simulink model "MATLAB_TEST"  (R2019b)
settings: Solver=FixedStepDiscrete  StartTime=0  StopTime=50  FixedStep=0.0025  RelTol=1e-3
undefined symbols (not defined in the file): BCM_COM_PROC_P20, BCM_COM_PROC_P20_SFW_R2018b, BCM_COM_PROC_P2_5, BCM_COM_PROC_P2_5_SFW_R2018b, BCM_COM_PROC_P5, BCM_COM_PROC_P5_SFW_R2018b, BCMA_ACCU_PT_Conf_Flt, BCMA_ACCU_PT_Unconf_Flt, BCMA_Antiskid_Off_Sanction, BCMA_Avionics_Conf_Flt, BCMA_BCM_CCDL_Conf_Flt, BCMA_BCM_CCDL_Unconf_Flt, BCMA_BCM_DBCU_INHIBITION_Conf_Flt, BCMA_BCM_DBCU_INHIBITION_Unconf_Flt, BCMA_BCP_ALT_Disp_Sw_Conf_Flt, BCMA_BCP_ALT_Disp_Sw_Unconf_Flt, BCMA_BCP_ALT_SW_ON_CMD_Conf_Flt, BCMA_BCP_ALT_SW_ON_CMD_Unconf_Flt, BCMA_BCP_PARK_OFF_SW_CMD_Conf_Flt, BCMA_BCP_PARK_OFF_SW_CMD_Unconf_Flt, BCMA_CF_BSELV_JCL, BCMA_CF_BSELV_JOP, BCMA_CF_BSELV_OC, BCMA_CF_BSELV_SC, BCMA_CF_LH_SV_JCL, BCMA_CF_LH_SV_JOP, BCMA_CF_LH_SV_OC, BCMA_CF_LH_SV_SC, BCMA_CF_PARK_BRK, BCMA_CF_RESIDUAL_PRESS, BCMA_CF_RH_SV_JCL, BCMA_CF_RH_SV_JOP, BCMA_CF_RH_SV_OC, BCMA_CF_RH_SV_SC, BCMA_CF_SELV_JCL, BCMA_CF_SELV_JOP, BCMA_CF_SELV_OC, BCMA_CF_SELV_SC, BCMA_CF_SV_DRIFT, BCMA_DBCU_ALT_MODE_Conf_Flt, BCMA_DBCU_ALT_MODE_Unconf_Flt, BCMA_DBCU_BRK_ORDER_FAIL_Conf_Flt, BCMA_DBCU_BRK_ORDER_FAIL_Unconf_Flt, BCMA_DBCU_Conf_Flt, BCMA_DBCU_DISPATCH_SW_ON_Conf_Flt, BCMA_DBCU_DISPATCH_SW_ON_Unconf_Flt, BCMA_DBCU_FAILED_Conf_Flt, BCMA_DBCU_FAILED_Unconf_Flt, BCMA_DFCS1_Capsule_Validity, BCMA_DFCS1_Label202_Corrupted, BCMA_DFCS1_Label202_Not_Refreshed, BCMA_DFCS1_Label204_Corrupted, BCMA_DFCS1_Label204_Not_Refreshed, BCMA_DFCS1_Label205_Corrupted, BCMA_DFCS1_Label205_Not_Refreshed, BCMA_DFCS1_Label206_Corrupted, BCMA_DFCS1_Label206_Not_Refreshed, BCMA_DFCS1_Label207_Corrupted, BCMA_DFCS1_Label207_Not_Refreshed, BCMA_DFCS3_Capsule_Validity ... (+762)
libraries: simulink x73, lib_MBD_Control x5
(part 12 of 16)

== system MATLAB_TEST/AVIONICS/Brake_Control_Module_Side_A/BCSA Controller CP/BCM_COM_PROC_P2_5/BCM_COM_PROC_P2_5 ==
  V_BCM_COM_Tacho_Acq_W12 : Inport
  V_BCM_COM_Tacho_Unconf_Flt_W12 : Inport  Port=2
  V_BCM_COM_Tacho_Conf_Flt_W12 : Inport  Port=3
  V_BCM_COM_Tacho_Acq_W34 : Inport  Port=4
  V_BCM_COM_Tacho_Unconf_Flt_W34 : Inport  Port=5
  V_BCM_COM_Tacho_Conf_Flt_W34 : Inport  Port=6
  V_BCM_COM_Whl_LP_AS_Curr_Order_W12 : Inport  Port=7
  V_BCM_COM_Press_Cmd_Rate_Lim : Inport  Port=8
  V_BCM_COM_Whl_LP_AS_Curr_Order_W34 : Inport  Port=9
  V_BCM_COM_Global_Reference_Spd : Inport  Port=10
  V_BCM_COM_Wheels_Global_Spun_Up_Ste : Inport  Port=11
  BCM_Tuning : Inport  Port=12
  BCM_COM_PROC_P2_5 : S-Function  FunctionName=BCM_COM_PROC_P2_5_SFCT  SFunctionModules=|  SFunctionDeploymentMode=off  EnableBusSupport=off
      | BCM_COM_PROC_P2_5
      | BCM_COM_PROC_P2_5_SFCT
      | AC_Accel_Computation
      | FilteredWheelSpeed
      | ComputeAcqTachoWheelSpeed
      | ComputeTachometerError
      | ComputeFilteredWheelSpeed
      | ComputeRateLimitedWheelSpeed
      | ComputeWheelSpeedPreFiltering
      | F_ASLIB_10
      | F_Interpolate_ASLIB
      | DERIV_ASLIB
      | Filter_Wheel_Speeds_Noise
      | F_WHEELSPEED_FILTERING_BCS_SCM_IWS_C1
      | IND_FilteredWheelSpeed_SCM_IWS_C1
      | ComputeRateLimitedWheelSpeed_SCM_IWS_C1
      | ComputeTachometerError_SCM_IWS_C1
      | ComputeAsFilteredWheelSpeed_SCM_IWS_C1
      | PBS1_ASLIB
      | ComputeAntiskidFilterTimeConstant_SCM_IWS_C1
      | LIM_ASLIB
      | ComputeFilteredWheelSpeed_SCM_IWS_C1
      | FILT_ASLIB
      | ComputeWheelSpeedPreFiltering_SCM_IWS_C1
      | MIN_ASLIB_float32
      | MAX_ASLIB_float32
      | MINMAX4_ASLIB_float32
      | ComputeAcqTachoWheelSpeed_SCM_IWS_C1
      | MEM_ASLIB_float32
      | Consolidate_Wheel_Speeds
      | F_WHEEL_SPEED_CONSOLIDATION_BCS_SCM_WSC_C1
      | ComputeWheelSpeedConsoFunction_SCM_WSC_C1
      | ComputeWheelSpeedConso_SCM_WSC_C1
      | AIG4_ASLIB_float32
      | ComputeTachometerValidity_SCM_WSC_C1
      | BCM_COM_PROC_P2_5_KCG66_kcg_types
      | BCM_COM_PROC_P2_5_KCG66_kcg_consts
      | BCM_COM_PROC_P2_5_KCG66_kcg_consts
  DTC{1,4,7..10} (6 alike) : DataTypeConversion  OutDataTypeStr=single  SaturateOnIntegerOverflow=on  RndMeth=Zero
  DTC{2..3,5..6,11} (5 alike) : DataTypeConversion  OutDataTypeStr=boolean  SaturateOnIntegerOverflow=on  RndMeth=Zero
  Prb_AntiskidFilterTimeConstant : Terminator
  Prb_AntiskidFilterTimeConstant (1) : Terminator
  Prb_AntiskidFilterTimeConstant (2) : Terminator
  Prb_AntiskidFilterTimeConstant (3) : Terminator
  Prb_FilteredWheelSpeedAverage : Terminator
  Prb_FilteredWheelSpeedAverage (1) : Terminator
  Prb_FilteredWheelSpeedAverage (2) : Terminator
  Prb_FilteredWheelSpeedAverage (3) : Terminator
  Prb_RateLimitedWheelSpeed : Terminator
  Prb_RateLimitedWheelSpeed (1) : Terminator
  Prb_RateLimitedWheelSpeed (2) : Terminator
  Prb_RateLimitedWheelSpeed (3) : Terminator
  Prb_TachometerError : Terminator
  Prb_TachometerError (1) : Terminator
  Prb_TachometerError (2) : Terminator
  Prb_TachometerError (3) : Terminator
  Prb_WheelSpeed : Terminator
  Prb_WheelSpeed (1) : Terminator
  Prb_WheelSpeed (2) : Terminator
  Prb_WheelSpeed (3) : Terminator
  Prb_WheelSpeedAverage : Terminator
  Prb_WheelSpeedAverage (1) : Terminator
  Prb_WheelSpeedAverage (2) : Terminator
  Prb_WheelSpeedAverage (3) : Terminator
  Prb_WheelSpeedMax4 : Terminator
  Prb_WheelSpeedMax4 (1) : Terminator
  Prb_WheelSpeedMax4 (2) : Terminator
  Prb_WheelSpeedMax4 (3) : Terminator
  Prb_WheelSpeedMin4 : Terminator
  Prb_WheelSpeedMin4 (1) : Terminator
  Prb_WheelSpeedMin4 (2) : Terminator
  Prb_WheelSpeedMin4 (3) : Terminator
  Prb_WhlSpdIntermediate : Terminator
  Prb_WhlSpdIntermediate (1) : Terminator
  Prb_WhlSpdIntermediate (2) : Terminator
  Prb_WhlSpdIntermediate (3) : Terminator
  Subsystem : Subsystem
  v_BCM_COM_Press_Cmd_Rate_Lim_W12 : Terminator
  v_BCM_COM_Press_Cmd_Rate_Lim_W34 : Terminator
  V_BCM_COM_Wheel_Speed_Cons_W12 : Outport
  V_BCM_COM_Wheel_Speed_W12 : Outport  Port=2
  V_BCM_COM_Wheel_Speed_Val_W12 : Outport  Port=3
  V_BCM_COM_Wheel_Speed_Cons_W34 : Outport  Port=4
  V_BCM_COM_Wheel_Speed_W34 : Outport  Port=5
  V_BCM_COM_Wheel_Speed_Val_W34 : Outport  Port=6
  V_BCM_COM_Whl_Filt_Spd_For_AS_W12 : Outport  Port=7
  V_BCM_COM_Wheel_Filtered_Speed_W12 : Outport  Port=8
  V_BCM_COM_Min_Last_8_Whl_Spd_W12 : Outport  Port=9
  V_BCM_COM_Max_Last_8_Whl_Spd_W12 : Outport  Port=10
  V_BCM_COM_Whl_Filt_Spd_For_AS_W34 : Outport  Port=11
  V_BCM_COM_Wheel_Filtered_Speed_W34 : Outport  Port=12
  V_BCM_COM_Min_Last_8_Whl_Spd_W34 : Outport  Port=13
  V_BCM_COM_Max_Last_8_Whl_Spd_W34 : Outport  Port=14
  V_BCM_COM_DCL_Acc : Outport  Port=15
  V_BCM_COM_CT_BCS_WS_First_Filter : Outport  Port=16
  wires:
  V_BCM_COM_Tacho_Acq_W12/1 -> DTC1/1
  DTC1/1 -> BCM_COM_PROC_P2_5/1
  V_BCM_COM_Tacho_Unconf_Flt_W12/1 -> DTC2/1
  DTC2/1 -> BCM_COM_PROC_P2_5/2
  V_BCM_COM_Tacho_Conf_Flt_W12/1 -> DTC3/1
  DTC3/1 -> BCM_COM_PROC_P2_5/3
  V_BCM_COM_Tacho_Acq_W34/1 -> DTC4/1
  DTC4/1 -> BCM_COM_PROC_P2_5/4
  V_BCM_COM_Tacho_Unconf_Flt_W34/1 -> DTC5/1
  DTC5/1 -> BCM_COM_PROC_P2_5/5
  V_BCM_COM_Tacho_Conf_Flt_W34/1 -> DTC6/1
  DTC6/1 -> BCM_COM_PROC_P2_5/6
  V_BCM_COM_Whl_LP_AS_Curr_Order_W12/1 -> DTC7/1
  DTC7/1 -> BCM_COM_PROC_P2_5/7
  V_BCM_COM_Press_Cmd_Rate_Lim/1 -> DTC8/1
  DTC8/1 -> BCM_COM_PROC_P2_5/8
  V_BCM_COM_Whl_LP_AS_Curr_Order_W34/1 -> DTC9/1
  DTC9/1 -> BCM_COM_PROC_P2_5/9
  V_BCM_COM_Global_Reference_Spd/1 -> DTC10/1
  DTC10/1 -> BCM_COM_PROC_P2_5/10
  V_BCM_COM_Wheels_Global_Spun_Up_Ste/1 -> DTC11/1
  DTC11/1 -> BCM_COM_PROC_P2_5/11
  BCM_COM_PROC_P2_5/1 -> V_BCM_COM_Wheel_Speed_Cons_W12/1
  BCM_COM_PROC_P2_5/2 -> V_BCM_COM_Wheel_Speed_W12/1
  BCM_COM_PROC_P2_5/3 -> V_BCM_COM_Wheel_Speed_Val_W12/1
  BCM_COM_PROC_P2_5/4 -> V_BCM_COM_Wheel_Speed_Cons_W34/1
  BCM_COM_PROC_P2_5/5 -> V_BCM_COM_Wheel_Speed_W34/1
  BCM_COM_PROC_P2_5/6 -> V_BCM_COM_Wheel_Speed_Val_W34/1
  BCM_COM_PROC_P2_5/7 -> V_BCM_COM_Whl_Filt_Spd_For_AS_W12/1
  BCM_COM_PROC_P2_5/8 -> V_BCM_COM_Wheel_Filtered_Speed_W12/1
  BCM_COM_PROC_P2_5/9 -> V_BCM_COM_Min_Last_8_Whl_Spd_W12/1
  BCM_COM_PROC_P2_5/10 -> V_BCM_COM_Max_Last_8_Whl_Spd_W12/1
  BCM_COM_PROC_P2_5/11 -> V_BCM_COM_Whl_Filt_Spd_For_AS_W34/1
  BCM_COM_PROC_P2_5/12 -> V_BCM_COM_Wheel_Filtered_Speed_W34/1
  BCM_COM_PROC_P2_5/13 -> V_BCM_COM_Min_Last_8_Whl_Spd_W34/1
  BCM_COM_PROC_P2_5/14 -> V_BCM_COM_Max_Last_8_Whl_Spd_W34/1
  BCM_COM_PROC_P2_5/15 -> V_BCM_COM_DCL_Acc/1
  BCM_COM_PROC_P2_5/16 -> V_BCM_COM_CT_BCS_WS_First_Filter/1
  BCM_COM_PROC_P2_5/17 -> Prb_WheelSpeed/1  "Prb_WheelSpeed_1_BCMA"
  BCM_COM_PROC_P2_5/18 -> Prb_WhlSpdIntermediate/1  "Prb_WhlSpdIntermediate_1_BCMA"
  BCM_COM_PROC_P2_5/19 -> Prb_WheelSpeedMin4/1  "Prb_WheelSpeedMin4_1_BCMA"
  BCM_COM_PROC_P2_5/20 -> Prb_WheelSpeedMax4/1  "Prb_WheelSpeedMax4_1_BCMA"
  BCM_COM_PROC_P2_5/21 -> Prb_WheelSpeedAverage/1  "Prb_WheelSpeedAverage_1_BCMA"
  BCM_COM_PROC_P2_5/22 -> Prb_FilteredWheelSpeedAverage/1  "Prb_FilteredWheelSpeedAverage_1_BCMA"
  BCM_COM_PROC_P2_5/23 -> Prb_TachometerError/1  "Prb_TachometerError_1_BCMA"
  BCM_COM_PROC_P2_5/24 -> Prb_RateLimitedWheelSpeed/1  "Prb_RateLimitedWheelSpeed_1_BCMA"
  BCM_COM_PROC_P2_5/25 -> Prb_AntiskidFilterTimeConstant/1  "Prb_AntiskidFilterTimeConstant_1_BCMA"
  BCM_COM_PROC_P2_5/26 -> Prb_WheelSpeed (1)/1  "Prb_WheelSpeed_2_BCMA"
  BCM_COM_PROC_P2_5/27 -> Prb_WhlSpdIntermediate (1)/1  "Prb_WhlSpdIntermediate_2_BCMA"
  BCM_COM_PROC_P2_5/28 -> Prb_WheelSpeedMin4 (1)/1  "Prb_WheelSpeedMin4_2_BCMA"
  BCM_COM_PROC_P2_5/29 -> Prb_WheelSpeedMax4 (1)/1  "Prb_WheelSpeedMax4_2_BCMA"
  BCM_COM_PROC_P2_5/30 -> Prb_WheelSpeedAverage (1)/1  "Prb_WheelSpeedAverage_2_BCMA"
  BCM_COM_PROC_P2_5/31 -> Prb_FilteredWheelSpeedAverage (1)/1  "Prb_FilteredWheelSpeedAverage_2_BCMA"
  BCM_COM_PROC_P2_5/32 -> Prb_TachometerError (1)/1  "Prb_TachometerError_2_BCMA"
  BCM_COM_PROC_P2_5/33 -> Prb_RateLimitedWheelSpeed (1)/1  "Prb_RateLimitedWheelSpeed_2_BCMA"
  BCM_COM_PROC_P2_5/34 -> Prb_AntiskidFilterTimeConstant (1)/1  "Prb_AntiskidFilterTimeConstant_2_BCMA"
  BCM_COM_PROC_P2_5/35 -> Prb_WheelSpeed (2)/1  "Prb_WheelSpeed_3_BCMA"
  BCM_COM_PROC_P2_5/36 -> Prb_WhlSpdIntermediate (2)/1  "Prb_WhlSpdIntermediate_3_BCMA"
  BCM_COM_PROC_P2_5/37 -> Prb_WheelSpeedMin4 (2)/1  "Prb_WheelSpeedMin4_3_BCMA"
  BCM_COM_PROC_P2_5/38 -> Prb_WheelSpeedMax4 (2)/1  "Prb_WheelSpeedMax4_3_BCMA"
  BCM_COM_PROC_P2_5/39 -> Prb_WheelSpeedAverage (2)/1  "Prb_WheelSpeedAverage_3_BCMA"
  BCM_COM_PROC_P2_5/40 -> Prb_FilteredWheelSpeedAverage (2)/1  "Prb_FilteredWheelSpeedAverage_3_BCMA"
  BCM_COM_PROC_P2_5/41 -> Prb_TachometerError (2)/1  "Prb_TachometerError_3_BCMA"
  BCM_COM_PROC_P2_5/42 -> Prb_RateLimitedWheelSpeed (2)/1  "Prb_RateLimitedWheelSpeed_3_BCMA"
  BCM_COM_PROC_P2_5/43 -> Prb_AntiskidFilterTimeConstant (2)/1  "Prb_AntiskidFilterTimeConstant_3_BCMA"
  BCM_COM_PROC_P2_5/44 -> Prb_WheelSpeed (3)/1  "Prb_WheelSpeed_4_BCMA"
  BCM_COM_PROC_P2_5/45 -> Prb_WhlSpdIntermediate (3)/1  "Prb_WhlSpdIntermediate_4_BCMA"
  BCM_COM_PROC_P2_5/46 -> Prb_WheelSpeedMin4 (3)/1  "Prb_WheelSpeedMin4_4_BCMA"
  BCM_COM_PROC_P2_5/47 -> Prb_WheelSpeedMax4 (3)/1  "Prb_WheelSpeedMax4_4_BCMA"
  BCM_COM_PROC_P2_5/48 -> Prb_WheelSpeedAverage (3)/1  "Prb_WheelSpeedAverage_4_BCMA"
  BCM_COM_PROC_P2_5/49 -> Prb_FilteredWheelSpeedAverage (3)/1  "Prb_FilteredWheelSpeedAverage_4_BCMA"
  BCM_COM_PROC_P2_5/50 -> Prb_TachometerError (3)/1  "Prb_TachometerError_4_BCMA"
  BCM_COM_PROC_P2_5/51 -> Prb_RateLimitedWheelSpeed (3)/1  "Prb_RateLimitedWheelSpeed_4_BCMA"
  BCM_COM_PROC_P2_5/52 -> Prb_AntiskidFilterTimeConstant (3)/1  "Prb_AntiskidFilterTimeConstant_4_BCMA"
  BCM_COM_PROC_P2_5/53 -> v_BCM_COM_Press_Cmd_Rate_Lim_W12/1  "v_BCM_COM_Press_Cmd_Rate_Lim_W12_1_BCMA"
  BCM_COM_PROC_P2_5/54 -> v_BCM_COM_Press_Cmd_Rate_Lim_W34/1  "v_BCM_COM_Press_Cmd_Rate_Lim_W34_1_BCMA"
  BCM_Tuning/1 -> Subsystem/1(In1)
  Subsystem/1(Out1) -> BCM_COM_PROC_P2_5/12
  Subsystem/2(Out2) -> BCM_COM_PROC_P2_5/13
  Subsystem/3(Out3) -> BCM_COM_PROC_P2_5/14
  Subsystem/4(Out4) -> BCM_COM_PROC_P2_5/15
  Subsystem/5(Out5) -> BCM_COM_PROC_P2_5/16
  Subsystem/6(Out6) -> BCM_COM_PROC_P2_5/17
  Subsystem/7(Out7) -> BCM_COM_PROC_P2_5/18
  Subsystem/8(Out8) -> BCM_COM_PROC_P2_5/19
  Subsystem/9(Out9) -> BCM_COM_PROC_P2_5/20
  Subsystem/10(Out10) -> BCM_COM_PROC_P2_5/21
  Subsystem/11(Out11) -> BCM_COM_PROC_P2_5/22
  Subsystem/12(Out12) -> BCM_COM_PROC_P2_5/23
  Subsystem/13(Out13) -> BCM_COM_PROC_P2_5/24
  Subsystem/14(Out14) -> BCM_COM_PROC_P2_5/25
  Subsystem/15(Out15) -> BCM_COM_PROC_P2_5/26
  Subsystem/16(Out16) -> BCM_COM_PROC_P2_5/27
  Subsystem/17(Out17) -> BCM_COM_PROC_P2_5/28
  Subsystem/18(Out18) -> BCM_COM_PROC_P2_5/29
  Subsystem/19(Out19) -> BCM_COM_PROC_P2_5/30
  Subsystem/20(Out20) -> BCM_COM_PROC_P2_5/31
  Subsystem/21(Out21) -> BCM_COM_PROC_P2_5/32
  Subsystem/22(Out22) -> BCM_COM_PROC_P2_5/33
  Subsystem/23(Out23) -> BCM_COM_PROC_P2_5/34
  Subsystem/24(Out24) -> BCM_COM_PROC_P2_5/35
  Subsystem/25(Out25) -> BCM_COM_PROC_P2_5/36

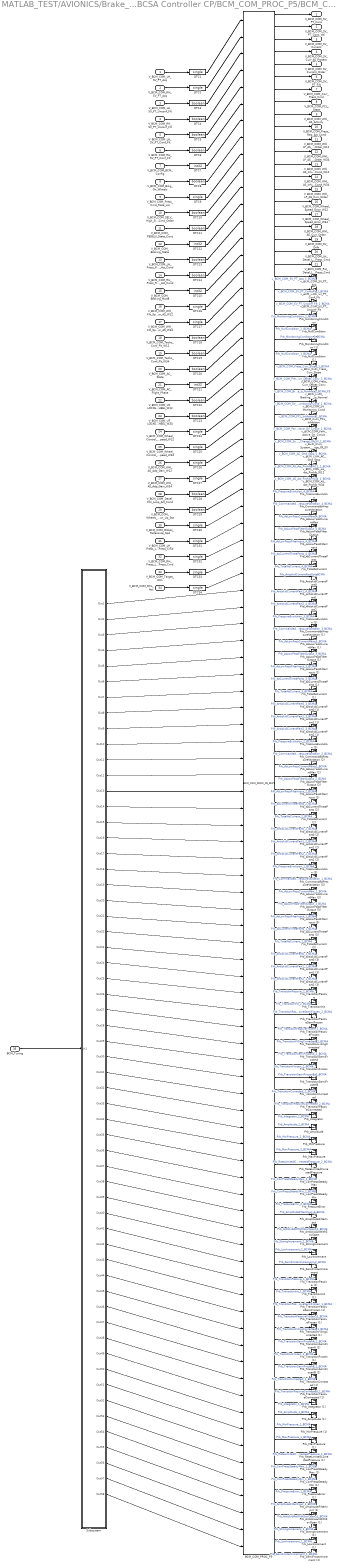
== system MATLAB_TEST/AVIONICS/Brake_Control_Module_Side_A/BCSA Controller CP/BCM_COM_PROC_P5/BCM_COM_PROC_P5 ==
  V_BCM_COM_LH_SV_PT_Acq : Inport
  V_BCM_COM_RH_SV_PT_Acq : Inport  Port=2
  V_BCM_COM_LH_SV_PT_Unconf_Flt : Inport  Port=3
  V_BCM_COM_RH_SV_PT_Unconf_Flt : Inport  Port=4
  V_BCM_COM_LH_SV_PT_Conf_Flt : Inport  Port=5
  V_BCM_COM_RH_SV_PT_Conf_Flt : Inport  Port=6
  V_BCM_COM_BCM_Config : Inport  Port=7
  V_BCM_COM_Brkg_On_Wheels : Inport  Port=8
  V_BCM_COM_Press_Cmd_Rate_Lim : Inport  Port=9
  V_BCM_COM_SELV_High_Side_Cmd_Order : Inport  Port=10
  V_BCM_COM_PBSELV_State_Cons : Inport  Port=11
  V_BCM_COM_Braking_State : Inport  Port=12
  V_BCM_COM_LH_Press_Reg_FT_Act_Cond : Inport  Port=13
  V_BCM_COM_RH_Press_Reg_FT_Act_Cond : Inport  Port=14
  V_BCM_COM_Braking_Mode : Inport  Port=15
  V_BCM_COM_Whl_Filt_Spd_For_AS_W12 : Inport  Port=16
  V_BCM_COM_Whl_Filt_Spd_For_AS_W34 : Inport  Port=17
  V_BCM_COM_Tacho_Conf_Flt_W12 : Inport  Port=18
  V_BCM_COM_Tacho_Conf_Flt_W34 : Inport  Port=19
  V_BCM_COM_AC_State : Inport  Port=20
  V_BCM_COM_AC_Flight_Phase : Inport  Port=21
  V_BCM_COM_UF_LOCKED_WHEEL_W12 : Inport  Port=22
  V_BCM_COM_UF_LOCKED_WHEEL_W34 : Inport  Port=23
  V_BCM_COM_Wheel_Control_Speed_W12 : Inport  Port=24
  V_BCM_COM_Wheel_Control_Speed_W34 : Inport  Port=25
  V_BCM_COM_Whl_AS_Adp_Gain_W12 : Inport  Port=26
  V_BCM_COM_Whl_AS_Adp_Gain_W34 : Inport  Port=27
  V_BCM_COM_Decel_Ctrl_Loop_Act_Cond : Inport  Port=28
  V_BCM_COM_Wheels_Global_Spun_Up_Ste : Inport  Port=29
  V_BCM_COM_Global_Reference_Spd : Inport  Port=30
  V_BCM_COM_LH_Press_Law_Brkg_Press_Cmd : Inport  Port=31
  V_BCM_COM_RH_Press_Law_Brkg_Press_Cmd : Inport  Port=32
  V_BCM_COM_Target_DCL : Inport  Port=33
  V_BCM_COM_DCL_Acc : Inport  Port=34
  BCM_Tuning : Inport  Port=35
  BCM_COM_PROC_P5 : S-Function  FunctionName=BCM_COM_PROC_P5_SFCT  SFunctionModules=<binary blob, 3799 chars, not shown>  SFunctionDeploymentMode=off  EnableBusSupport=off
  DTC{1..2,9,16..17,24..27,30..34} (14 alike) : DataTypeConversion  OutDataTypeStr=single  SaturateOnIntegerOverflow=on  RndMeth=Zero
  DTC{3..6,8,10..11,13..14,18..20,22..23,28..29} (16 alike) : DataTypeConversion  OutDataTypeStr=boolean  SaturateOnIntegerOverflow=on  RndMeth=Zero
  DTC{7,12,15,21} (4 alike) : DataTypeConversion  OutDataTypeStr=int32  SaturateOnIntegerOverflow=on  RndMeth=Zero
  Prb_Amplitude : Terminator
  Prb_Amplitude (1) : Terminator
  Prb_AmplitudeFilterInput : Terminator
  Prb_AmplitudeFilterInput (1) : Terminator
  Prb_AntiskidActWithSovOpen : Terminator
  Prb_AntiskidActWithSovOpen (1) : Terminator
  Prb_AntiskidCurrentPart0 : Terminator
  Prb_AntiskidCurrentPart0 (1) : Terminator
  Prb_AntiskidCurrentPart0 (2) : Terminator
  Prb_AntiskidCurrentPart0 (3) : Terminator
  Prb_AntiskidCurrentPart1 : Terminator
  Prb_AntiskidCurrentPart1 (1) : Terminator
  Prb_AntiskidCurrentPart1 (2) : Terminator
  Prb_AntiskidCurrentPart1 (3) : Terminator
  Prb_AntiskidCurrentPart2 : Terminator
  Prb_AntiskidCurrentPart2 (1) : Terminator
  Prb_AntiskidCurrentPart2 (2) : Terminator
  Prb_AntiskidCurrentPart2 (3) : Terminator
  Prb_AsCurrentThreeParts : Terminator
  Prb_AsCurrentThreeParts (1) : Terminator
  Prb_AsCurrentThreeParts (2) : Terminator
  Prb_AsCurrentThreeParts (3) : Terminator
  Prb_AsLowPassCurrentMax : Terminator
  Prb_AsLowPassCurrentMax (1) : Terminator
  Prb_AsLowPassCurrentMax (2) : Terminator
  Prb_AsLowPassCurrentMax (3) : Terminator
  Prb_AsLowPassFilterInput : Terminator
  Prb_AsLowPassFilterInput (1) : Terminator
  Prb_AsLowPassFilterInput (2) : Terminator
  Prb_AsLowPassFilterInput (3) : Terminator
  Prb_AsLowPassFilterOutput : Terminator
  Prb_AsLowPassFilterOutput (1) : Terminator
  Prb_AsLowPassFilterOutput (2) : Terminator
  Prb_AsLowPassFilterOutput (3) : Terminator
  Prb_CommandedPressureVariation : Terminator
  Prb_CommandedPressureVariation (1) : Terminator
  Prb_CommandedPressureVariation (2) : Terminator
  Prb_CommandedPressureVariation (3) : Terminator
  Prb_CorrPressSteadyMax : Terminator
  Prb_CorrPressSteadyMax (1) : Terminator
  Prb_CorrPressSteadyMin : Terminator
  Prb_CorrPressSteadyMin (1) : Terminator
  Prb_Integrator : Terminator
  Prb_Integrator (1) : Terminator
  Prb_LowIncrement : Terminator
  Prb_LowIncrement (1) : Terminator
  Prb_MaxPressure : Terminator
  Prb_MaxPressure (1) : Terminator
  Prb_MinPressure : Terminator
  Prb_MinPressure (1) : Terminator
  Prb_MonitoringCondition : Terminator
  Prb_MonitoringCondition (1) : Terminator
  Prb_NullCondition : Terminator
  Prb_NullCondition (1) : Terminator
  Prb_PressureError : Terminator
  Prb_PressureError (1) : Terminator
  Prb_PressureEvolution : Terminator
  Prb_PressureEvolution (1) : Terminator
  Prb_PressureEvolution (2) : Terminator
  Prb_PressureEvolution (3) : Terminator
  Prb_RateLimitedCorrectedPressure : Terminator
  Prb_RateLimitedCorrectedPressure (1) : Terminator
  Prb_SemiFrozenIncrement : Terminator
  Prb_SemiFrozenIncrement (1) : Terminator
  Prb_StrongIncrement : Terminator
  Prb_StrongIncrement (1) : Terminator
  Prb_TotalAsCurrent : Terminator
  Prb_TotalAsCurrent (1) : Terminator
  Prb_TotalAsCurrent (2) : Terminator
  Prb_TotalAsCurrent (3) : Terminator
  Prb_TransitionCorrected : Terminator
  Prb_TransitionCorrected (1) : Terminator
  Prb_TransitionFillingCorrected : Terminator
  Prb_TransitionFillingCorrected (1) : Terminator
  Prb_TransitionFrozen : Terminator
  Prb_TransitionFrozen (1) : Terminator
  Prb_TransitionInit : Terminator
  Prb_TransitionInit (1) : Terminator
  Prb_TransitionPassive : Terminator
  Prb_TransitionPassive (1) : Terminator
  Prb_TransitionPassiveCorrrected : Terminator
  Prb_TransitionPassiveCorrrected (1) : Terminator
  Prb_TransitionPassiveFrozen : Terminator
  Prb_TransitionPassiveFrozen (1) : Terminator
  Prb_TransitionPassiveSemiFrozen : Terminator
  Prb_TransitionPassiveSemiFrozen (1) : Terminator
  Prb_TransitionSemiFrozenA : Terminator
  Prb_TransitionSemiFrozenA (1) : Terminator
  Prb_TransitionSemiFrozenB : Terminator
  Prb_TransitionSemiFrozenB (1) : Terminator
  Subsystem : Subsystem
  v_BCM_COM_AC_Gnd_Stop : Terminator
  v_BCM_COM_AS_Act_Prohib_W12 : Terminator
  v_BCM_COM_AS_Act_Prohib_W34 : Terminator
  v_BCM_COM_Braking_Ste_Is_Normal : Terminator
  v_BCM_COM_PCL_Inhibition : Terminator
  v_BCM_COM_Park_Active_On_Circuit : Terminator
  v_BCM_COM_Press_Curr_Offset_Conv : Terminator
  v_BCM_COM_Press_Curr_Slope : Terminator
  v_BCM_COM_SV_Monitoring_Cond : Terminator
  v_BCM_COM_SV_PT_Acq : Terminator
  v_BCM_COM_SV_PT_Conf_Flt : Terminator
  v_BCM_COM_SV_PT_Unconf_Flt : Terminator
  v_BCM_COM_System_In_Charge_Of_SV : Terminator
  V_BCM_COM_SV_PT_Cons : Outport
  V_BCM_COM_SV_PT_Cons_Val : Outport  Port=2
  V_BCM_COM_SV_Current : Outport  Port=3
  V_BCM_COM_SV_Curr_AS_Protect : Outport  Port=4
  V_BCM_COM_SV_Current_Order : Outport  Port=5
  V_BCM_COM_SV_PT_Filt : Outport  Port=6
  V_BCM_COM_Corr_Press_Cmd : Outport  Port=7
  V_BCM_COM_PCL_State : Outport  Port=8
  V_BCM_COM_Whl_AS_Activity : Outport  Port=9
  V_BCM_COM_Press_Reg_Act_Cond : Outport  Port=10
  V_BCM_COM_Whl_LP_AS_Curr_Order_W12 : Outport  Port=11
  V_BCM_COM_Whl_LP_AS_Curr_Order_W34 : Outport  Port=12
  V_BCM_COM_Whl_AS_Inhib_Cond_W12 : Outport  Port=13
  V_BCM_COM_Whl_AS_Inhib_Cond_W34 : Outport  Port=14
  V_BCM_COM_Whl_LP_AS_Curr_Order : Outport  Port=15
  V_BCM_COM_Wheel_Speed_Error_W12 : Outport  Port=16
  V_BCM_COM_Wheel_Speed_Error_W34 : Outport  Port=17
  V_BCM_COM_Whl_AS_Curr_Order : Outport  Port=18
  V_BCM_COM_SV_Drift : Outport  Port=19
  V_BCM_COM_LH_Decel_Law_Brkg_Press_Cmd : Outport  Port=20
  V_BCM_COM_RH_Decel_Law_Brkg_Press_Cmd : Outport  Port=21
  wires:
  BCM_COM_PROC_P5/124 -> Prb_SemiFrozenIncrement (1)/1  "Prb_SemiFrozenIncrement_1_BCMA"
  BCM_COM_PROC_P5/123 -> Prb_LowIncrement (1)/1  "Prb_LowIncrement_1_BCMA"
  BCM_COM_PROC_P5/122 -> Prb_StrongIncrement (1)/1  "Prb_StrongIncrement_1_BCMA"
  BCM_COM_PROC_P5/121 -> Prb_AntiskidActWithSovOpen (1)/1  "Prb_AntiskidActWithSovOpen_1_BCMA"
  BCM_COM_PROC_P5/120 -> Prb_AmplitudeFilterInput (1)/1  "Prb_AmplitudeFilterInput_1_BCMA"
  BCM_COM_PROC_P5/119 -> Prb_PressureError (1)/1  "Prb_PressureError_1_BCMA"
  BCM_COM_PROC_P5/118 -> Prb_CorrPressSteadyMin (1)/1  "Prb_CorrPressSteadyMin_1_BCMA"
  BCM_COM_PROC_P5/117 -> Prb_CorrPressSteadyMax (1)/1  "Prb_CorrPressSteadyMax_1_BCMA"
  BCM_COM_PROC_P5/116 -> Prb_RateLimitedCorrectedPressure (1)/1  "Prb_RateLimitedCorrectedPressure_1_BCMA"
  BCM_COM_PROC_P5/115 -> Prb_MaxPressure (1)/1  "Prb_MaxPressure_1_BCMA"
  BCM_COM_PROC_P5/114 -> Prb_MinPressure (1)/1  "Prb_MinPressure_1_BCMA"
  BCM_COM_PROC_P5/113 -> Prb_Amplitude (1)/1  "Prb_Amplitude_1_BCMA"
  BCM_COM_PROC_P5/112 -> Prb_Integrator (1)/1  "Prb_Integrator_1_BCMA"
  BCM_COM_PROC_P5/111 -> Prb_TransitionPassiveCorrrected (1)/1  "Prb_TransitionPassiveCorrrected_1_BCMA"
  BCM_COM_PROC_P5/110 -> Prb_TransitionCorrected (1)/1  "Prb_TransitionCorrected_1_BCMA"
  BCM_COM_PROC_P5/109 -> Prb_TransitionSemiFrozenB (1)/1  "Prb_TransitionSemiFrozenB_1_BCMA"
  BCM_COM_PROC_P5/108 -> Prb_TransitionFrozen (1)/1  "Prb_TransitionFrozen_1_BCMA"
  BCM_COM_PROC_P5/107 -> Prb_TransitionSemiFrozenA (1)/1  "Prb_TransitionSemiFrozenA_1_BCMA"
  BCM_COM_PROC_P5/106 -> Prb_TransitionFillingCorrected (1)/1  "Prb_TransitionFillingCorrected_1_BCMA"
  BCM_COM_PROC_P5/105 -> Prb_TransitionPassiveFrozen (1)/1  "Prb_TransitionPassiveFrozen_1_BCMA"
  BCM_COM_PROC_P5/104 -> Prb_TransitionPassiveSemiFrozen (1)/1  "Prb_TransitionPassiveSemiFrozen_1_BCMA"
  BCM_COM_PROC_P5/103 -> Prb_TransitionInit (1)/1  "Prb_TransitionInit_1_BCMA"
  BCM_COM_PROC_P5/102 -> Prb_TransitionPassive (1)/1  "Prb_TransitionPassive_1_BCMA"
  BCM_COM_PROC_P5/101 -> Prb_SemiFrozenIncrement/1  "Prb_SemiFrozenIncrement_2_BCMA"
  BCM_COM_PROC_P5/100 -> Prb_LowIncrement/1  "Prb_LowIncrement_2_BCMA"
  BCM_COM_PROC_P5/99 -> Prb_StrongIncrement/1  "Prb_StrongIncrement_2_BCMA"
  BCM_COM_PROC_P5/98 -> Prb_AntiskidActWithSovOpen/1  "Prb_AntiskidActWithSovOpen_2_BCMA"
  BCM_COM_PROC_P5/97 -> Prb_AmplitudeFilterInput/1  "Prb_AmplitudeFilterInput_2_BCMA"
  BCM_COM_PROC_P5/96 -> Prb_PressureError/1  "Prb_PressureError_2_BCMA"
  BCM_COM_PROC_P5/95 -> Prb_CorrPressSteadyMin/1  "Prb_CorrPressSteadyMin_2_BCMA"
  BCM_COM_PROC_P5/94 -> Prb_CorrPressSteadyMax/1  "Prb_CorrPressSteadyMax_2_BCMA"
  BCM_COM_PROC_P5/93 -> Prb_RateLimitedCorrectedPressure/1  "Prb_RateLimitedCorrectedPressure_2_BCMA"
  BCM_COM_PROC_P5/92 -> Prb_MaxPressure/1  "Prb_MaxPressure_2_BCMA"
  BCM_COM_PROC_P5/91 -> Prb_MinPressure/1  "Prb_MinPressure_2_BCMA"
  BCM_COM_PROC_P5/90 -> Prb_Amplitude/1  "Prb_Amplitude_2_BCMA"
  BCM_COM_PROC_P5/89 -> Prb_Integrator/1  "Prb_Integrator_2_BCMA"
  BCM_COM_PROC_P5/88 -> Prb_TransitionPassiveCorrrected/1  "Prb_TransitionPassiveCorrrected_2_BCMA"
  BCM_COM_PROC_P5/87 -> Prb_TransitionCorrected/1  "Prb_TransitionCorrected_2_BCMA"
  BCM_COM_PROC_P5/86 -> Prb_TransitionSemiFrozenB/1  "Prb_TransitionSemiFrozenB_2_BCMA"
  BCM_COM_PROC_P5/85 -> Prb_TransitionFrozen/1  "Prb_TransitionFrozen_2_BCMA"
  BCM_COM_PROC_P5/84 -> Prb_TransitionSemiFrozenA/1  "Prb_TransitionSemiFrozenA_2_BCMA"
  BCM_COM_PROC_P5/83 -> Prb_TransitionFillingCorrected/1  "Prb_TransitionFillingCorrected_2_BCMA"
  BCM_COM_PROC_P5/82 -> Prb_TransitionPassiveFrozen/1  "Prb_TransitionPassiveFrozen_2_BCMA"
  BCM_COM_PROC_P5/81 -> Prb_TransitionPassiveSemiFrozen/1  "Prb_TransitionPassiveSemiFrozen_2_BCMA"
  BCM_COM_PROC_P5/80 -> Prb_TransitionInit/1  "Prb_TransitionInit_2_BCMA"
  BCM_COM_PROC_P5/79 -> Prb_TransitionPassive/1  "Prb_TransitionPassive_2_BCMA"
  BCM_COM_PROC_P5/78 -> Prb_AntiskidCurrentPart2 (3)/1  "Prb_AntiskidCurrentPart2_1_BCMA"
  BCM_COM_PROC_P5/77 -> Prb_AntiskidCurrentPart1 (3)/1  "Prb_AntiskidCurrentPart1_1_BCMA"
  BCM_COM_PROC_P5/76 -> Prb_AntiskidCurrentPart0 (3)/1  "Prb_AntiskidCurrentPart0_1_BCMA"
  BCM_COM_PROC_P5/75 -> Prb_TotalAsCurrent (3)/1  "Prb_TotalAsCurrent_1_BCMA"
  BCM_COM_PROC_P5/74 -> Prb_AsCurrentThreeParts (3)/1  "Prb_AsCurrentThreeParts_1_BCMA"
  BCM_COM_PROC_P5/73 -> Prb_AsLowPassFilterInput (3)/1  "Prb_AsLowPassFilterInput_1_BCMA"
  BCM_COM_PROC_P5/72 -> Prb_AsLowPassFilterOutput (3)/1  "Prb_AsLowPassFilterOutput_1_BCMA"
  BCM_COM_PROC_P5/71 -> Prb_AsLowPassCurrentMax (3)/1  "Prb_AsLowPassCurrentMax_1_BCMA"
  BCM_COM_PROC_P5/70 -> Prb_CommandedPressureVariation (3)/1  "Prb_CommandedPressureVariation_1_BCMA"
  BCM_COM_PROC_P5/69 -> Prb_PressureEvolution (3)/1  "Prb_PressureEvolution_1_BCMA"
  BCM_COM_PROC_P5/68 -> Prb_AntiskidCurrentPart2 (2)/1  "Prb_AntiskidCurrentPart2_2_BCMA"
  BCM_COM_PROC_P5/67 -> Prb_AntiskidCurrentPart1 (2)/1  "Prb_AntiskidCurrentPart1_2_BCMA"
  BCM_COM_PROC_P5/66 -> Prb_AntiskidCurrentPart0 (2)/1  "Prb_AntiskidCurrentPart0_2_BCMA"
  BCM_COM_PROC_P5/65 -> Prb_TotalAsCurrent (2)/1  "Prb_TotalAsCurrent_2_BCMA"
  BCM_COM_PROC_P5/64 -> Prb_AsCurrentThreeParts (2)/1  "Prb_AsCurrentThreeParts_2_BCMA"
  BCM_COM_PROC_P5/63 -> Prb_AsLowPassFilterInput (2)/1  "Prb_AsLowPassFilterInput_2_BCMA"
  BCM_COM_PROC_P5/62 -> Prb_AsLowPassFilterOutput (2)/1  "Prb_AsLowPassFilterOutput_2_BCMA"
  BCM_COM_PROC_P5/61 -> Prb_AsLowPassCurrentMax (2)/1  "Prb_AsLowPassCurrentMax_2_BCMA"
  BCM_COM_PROC_P5/60 -> Prb_CommandedPressureVariation (2)/1  "Prb_CommandedPressureVariation_2_BCMA"
  BCM_COM_PROC_P5/59 -> Prb_PressureEvolution (2)/1  "Prb_PressureEvolution_2_BCMA"
  BCM_COM_PROC_P5/58 -> Prb_AntiskidCurrentPart2 (1)/1  "Prb_AntiskidCurrentPart2_3_BCMA"
  BCM_COM_PROC_P5/57 -> Prb_AntiskidCurrentPart1 (1)/1  "Prb_AntiskidCurrentPart1_3_BCMA"
  BCM_COM_PROC_P5/56 -> Prb_AntiskidCurrentPart0 (1)/1  "Prb_AntiskidCurrentPart0_3_BCMA"
  BCM_COM_PROC_P5/55 -> Prb_TotalAsCurrent (1)/1  "Prb_TotalAsCurrent_3_BCMA"
  BCM_COM_PROC_P5/54 -> Prb_AsCurrentThreeParts (1)/1  "Prb_AsCurrentThreeParts_3_BCMA"
  BCM_COM_PROC_P5/53 -> Prb_AsLowPassFilterInput (1)/1  "Prb_AsLowPassFilterInput_3_BCMA"
  BCM_COM_PROC_P5/52 -> Prb_AsLowPassFilterOutput (1)/1  "Prb_AsLowPassFilterOutput_3_BCMA"
  BCM_COM_PROC_P5/51 -> Prb_AsLowPassCurrentMax (1)/1  "Prb_AsLowPassCurrentMax_3_BCMA"
  BCM_COM_PROC_P5/50 -> Prb_CommandedPressureVariation (1)/1  "Prb_CommandedPressureVariation_3_BCMA"
  BCM_COM_PROC_P5/49 -> Prb_PressureEvolution (1)/1  "Prb_PressureEvolution_3_BCMA"
  BCM_COM_PROC_P5/48 -> Prb_AntiskidCurrentPart2/1  "Prb_AntiskidCurrentPart2_4_BCMA"
  BCM_COM_PROC_P5/47 -> Prb_AntiskidCurrentPart1/1  "Prb_AntiskidCurrentPart1_4_BCMA"
  BCM_COM_PROC_P5/46 -> Prb_AntiskidCurrentPart0/1  "Prb_AntiskidCurrentPart0_4_BCMA"
  BCM_COM_PROC_P5/45 -> Prb_TotalAsCurrent/1  "Prb_TotalAsCurrent_4_BCMA"
  BCM_COM_PROC_P5/44 -> Prb_AsCurrentThreeParts/1  "Prb_AsCurrentThreeParts_4_BCMA"
  BCM_COM_PROC_P5/43 -> Prb_AsLowPassFilterInput/1  "Prb_AsLowPassFilterInput_4_BCMA"
  BCM_COM_PROC_P5/42 -> Prb_AsLowPassFilterOutput/1  "Prb_AsLowPassFilterOutput_4_BCMA"
  BCM_COM_PROC_P5/41 -> Prb_AsLowPassCurrentMax/1  "Prb_AsLowPassCurrentMax_4_BCMA"
  BCM_COM_PROC_P5/40 -> Prb_CommandedPressureVariation/1  "Prb_CommandedPressureVariation_4_BCMA"
  BCM_COM_PROC_P5/39 -> Prb_PressureEvolution/1  "Prb_PressureEvolution_4_BCMA"
  BCM_COM_PROC_P5/38 -> v_BCM_COM_AS_Act_Prohib_W34/1  "v_BCM_COM_AS_Act_Prohib_W34_1_BCMA"
  BCM_COM_PROC_P5/37 -> v_BCM_COM_AS_Act_Prohib_W12/1  "v_BCM_COM_AS_Act_Prohib_W12_1_BCMA"
  BCM_COM_PROC_P5/36 -> v_BCM_COM_AC_Gnd_Stop/1  "v_BCM_COM_AC_Gnd_Stop_1_BCMA"
  BCM_COM_PROC_P5/35 -> v_BCM_COM_System_In_Charge_Of_SV/1  "v_BCM_COM_System_In_Charge_Of_SV_1_BCMA"
  BCM_COM_PROC_P5/34 -> v_BCM_COM_Park_Active_On_Circuit/1  "v_BCM_COM_Park_Active_On_Circuit_1_BCMA"
  BCM_COM_PROC_P5/33 -> v_BCM_COM_PCL_Inhibition/1  "v_BCM_COM_PCL_Inhibition_1_BCMA"
  BCM_COM_PROC_P5/32 -> v_BCM_COM_SV_Monitoring_Cond/1  "v_BCM_COM_SV_Monitoring_Cond_1_BCMA"
  BCM_COM_PROC_P5/31 -> v_BCM_COM_Braking_Ste_Is_Normal/1  "v_BCM_COM_Braking_Ste_Is_Normal_1_BCMA_P5"
  BCM_COM_PROC_P5/30 -> v_BCM_COM_Press_Curr_Offset_Conv/1  "v_BCM_COM_Press_Curr_Offset_Conv_1_BCMA"
  BCM_COM_PROC_P5/29 -> v_BCM_COM_Press_Curr_Slope/1  "v_BCM_COM_Press_Curr_Slope_1_BCMA"
  BCM_COM_PROC_P5/28 -> Prb_NullCondition (1)/1  "Prb_NullCondition_1_BCMA"
  BCM_COM_PROC_P5/27 -> Prb_MonitoringCondition (1)/1  "Prb_MonitoringCondition_1_BCMA"
  BCM_COM_PROC_P5/26 -> Prb_NullCondition/1  "Prb_NullCondition_2_BCMA"
  BCM_COM_PROC_P5/25 -> Prb_MonitoringCondition/1  "Prb_MonitoringCondition_2_BCMA"
  BCM_COM_PROC_P5/24 -> v_BCM_COM_SV_PT_Unconf_Flt/1  "v_BCM_COM_SV_PT_Unconf_Flt_1_BCMA"
  BCM_COM_PROC_P5/23 -> v_BCM_COM_SV_PT_Conf_Flt/1  "v_BCM_COM_SV_PT_Conf_Flt_1_BCMA"
  BCM_COM_PROC_P5/22 -> v_BCM_COM_SV_PT_Acq/1  "v_BCM_COM_SV_PT_Acq_1_BCMA"
  BCM_COM_PROC_P5/21 -> V_BCM_COM_RH_Decel_Law_Brkg_Press_Cmd/1
  BCM_COM_PROC_P5/20 -> V_BCM_COM_LH_Decel_Law_Brkg_Press_Cmd/1
  BCM_COM_PROC_P5/19 -> V_BCM_COM_SV_Drift/1
  BCM_COM_PROC_P5/18 -> V_BCM_COM_Whl_AS_Curr_Order/1
  BCM_COM_PROC_P5/17 -> V_BCM_COM_Wheel_Speed_Error_W34/1
  BCM_COM_PROC_P5/16 -> V_BCM_COM_Wheel_Speed_Error_W12/1
  BCM_COM_PROC_P5/15 -> V_BCM_COM_Whl_LP_AS_Curr_Order/1
  BCM_COM_PROC_P5/14 -> V_BCM_COM_Whl_AS_Inhib_Cond_W34/1
  BCM_COM_PROC_P5/13 -> V_BCM_COM_Whl_AS_Inhib_Cond_W12/1
  BCM_COM_PROC_P5/12 -> V_BCM_COM_Whl_LP_AS_Curr_Order_W34/1
  BCM_COM_PROC_P5/11 -> V_BCM_COM_Whl_LP_AS_Curr_Order_W12/1
  BCM_COM_PROC_P5/10 -> V_BCM_COM_Press_Reg_Act_Cond/1
  BCM_COM_PROC_P5/9 -> V_BCM_COM_Whl_AS_Activity/1
  BCM_COM_PROC_P5/8 -> V_BCM_COM_PCL_State/1
  BCM_COM_PROC_P5/7 -> V_BCM_COM_Corr_Press_Cmd/1
  BCM_COM_PROC_P5/6 -> V_BCM_COM_SV_PT_Filt/1
  BCM_COM_PROC_P5/5 -> V_BCM_COM_SV_Current_Order/1
  BCM_COM_PROC_P5/4 -> V_BCM_COM_SV_Curr_AS_Protect/1
  BCM_COM_PROC_P5/3 -> V_BCM_COM_SV_Current/1
  BCM_COM_PROC_P5/2 -> V_BCM_COM_SV_PT_Cons_Val/1
  BCM_COM_PROC_P5/1 -> V_BCM_COM_SV_PT_Cons/1
  DTC34/1 -> BCM_COM_PROC_P5/34
  V_BCM_COM_DCL_Acc/1 -> DTC34/1
  DTC33/1 -> BCM_COM_PROC_P5/33
  V_BCM_COM_Target_DCL/1 -> DTC33/1
  DTC32/1 -> BCM_COM_PROC_P5/32
  V_BCM_COM_RH_Press_Law_Brkg_Press_Cmd/1 -> DTC32/1
  DTC31/1 -> BCM_COM_PROC_P5/31
  V_BCM_COM_LH_Press_Law_Brkg_Press_Cmd/1 -> DTC31/1
  DTC30/1 -> BCM_COM_PROC_P5/30
  V_BCM_COM_Global_Reference_Spd/1 -> DTC30/1
  DTC29/1 -> BCM_COM_PROC_P5/29
  V_BCM_COM_Wheels_Global_Spun_Up_Ste/1 -> DTC29/1
  DTC28/1 -> BCM_COM_PROC_P5/28
  V_BCM_COM_Decel_Ctrl_Loop_Act_Cond/1 -> DTC28/1
  DTC27/1 -> BCM_COM_PROC_P5/27
  V_BCM_COM_Whl_AS_Adp_Gain_W34/1 -> DTC27/1
  DTC26/1 -> BCM_COM_PROC_P5/26
  V_BCM_COM_Whl_AS_Adp_Gain_W12/1 -> DTC26/1
  DTC25/1 -> BCM_COM_PROC_P5/25
  V_BCM_COM_Wheel_Control_Speed_W34/1 -> DTC25/1
  DTC24/1 -> BCM_COM_PROC_P5/24
  V_BCM_COM_Wheel_Control_Speed_W12/1 -> DTC24/1
  DTC23/1 -> BCM_COM_PROC_P5/23
  V_BCM_COM_UF_LOCKED_WHEEL_W34/1 -> DTC23/1
  DTC22/1 -> BCM_COM_PROC_P5/22
  V_BCM_COM_UF_LOCKED_WHEEL_W12/1 -> DTC22/1
  DTC21/1 -> BCM_COM_PROC_P5/21
  V_BCM_COM_AC_Flight_Phase/1 -> DTC21/1
  DTC20/1 -> BCM_COM_PROC_P5/20
  V_BCM_COM_AC_State/1 -> DTC20/1
  DTC19/1 -> BCM_COM_PROC_P5/19
  V_BCM_COM_Tacho_Conf_Flt_W34/1 -> DTC19/1
  DTC18/1 -> BCM_COM_PROC_P5/18
  V_BCM_COM_Tacho_Conf_Flt_W12/1 -> DTC18/1
  DTC17/1 -> BCM_COM_PROC_P5/17
  V_BCM_COM_Whl_Filt_Spd_For_AS_W34/1 -> DTC17/1
  DTC16/1 -> BCM_COM_PROC_P5/16
  V_BCM_COM_Whl_Filt_Spd_For_AS_W12/1 -> DTC16/1
  DTC15/1 -> BCM_COM_PROC_P5/15
  V_BCM_COM_Braking_Mode/1 -> DTC15/1
  DTC14/1 -> BCM_COM_PROC_P5/14
  V_BCM_COM_RH_Press_Reg_FT_Act_Cond/1 -> DTC14/1
  DTC13/1 -> BCM_COM_PROC_P5/13
  V_BCM_COM_LH_Press_Reg_FT_Act_Cond/1 -> DTC13/1
  DTC12/1 -> BCM_COM_PROC_P5/12
  V_BCM_COM_Braking_State/1 -> DTC12/1
  DTC11/1 -> BCM_COM_PROC_P5/11
  V_BCM_COM_PBSELV_State_Cons/1 -> DTC11/1
  DTC10/1 -> BCM_COM_PROC_P5/10
  V_BCM_COM_SELV_High_Side_Cmd_Order/1 -> DTC10/1
  DTC9/1 -> BCM_COM_PROC_P5/9
  V_BCM_COM_Press_Cmd_Rate_Lim/1 -> DTC9/1
  DTC8/1 -> BCM_COM_PROC_P5/8
  V_BCM_COM_Brkg_On_Wheels/1 -> DTC8/1
  DTC7/1 -> BCM_COM_PROC_P5/7
  V_BCM_COM_BCM_Config/1 -> DTC7/1
  DTC6/1 -> BCM_COM_PROC_P5/6
  V_BCM_COM_RH_SV_PT_Conf_Flt/1 -> DTC6/1
  DTC5/1 -> BCM_COM_PROC_P5/5
  V_BCM_COM_LH_SV_PT_Conf_Flt/1 -> DTC5/1
  DTC4/1 -> BCM_COM_PROC_P5/4
  V_BCM_COM_RH_SV_PT_Unconf_Flt/1 -> DTC4/1
  DTC3/1 -> BCM_COM_PROC_P5/3
  V_BCM_COM_LH_SV_PT_Unconf_Flt/1 -> DTC3/1
  DTC2/1 -> BCM_COM_PROC_P5/2
  V_BCM_COM_RH_SV_PT_Acq/1 -> DTC2/1
  DTC1/1 -> BCM_COM_PROC_P5/1
  V_BCM_COM_LH_SV_PT_Acq/1 -> DTC1/1
  BCM_Tuning/1 -> Subsystem/1(In1)
  Subsystem/1(Out1) -> BCM_COM_PROC_P5/35
  Subsystem/2(Out2) -> BCM_COM_PROC_P5/36
  Subsystem/3(Out3) -> BCM_COM_PROC_P5/37
  Subsystem/4(Out4) -> BCM_COM_PROC_P5/38
  Subsystem/5(Out5) -> BCM_COM_PROC_P5/39
  Subsystem/6(Out6) -> BCM_COM_PROC_P5/40
  Subsystem/7(Out7) -> BCM_COM_PROC_P5/41
  Subsystem/8(Out8) -> BCM_COM_PROC_P5/42
  Subsystem/9(Out9) -> BCM_COM_PROC_P5/43
  Subsystem/10(Out10) -> BCM_COM_PROC_P5/44
  Subsystem/11(Out11) -> BCM_COM_PROC_P5/45
  Subsystem/12(Out12) -> BCM_COM_PROC_P5/46
  Subsystem/13(Out13) -> BCM_COM_PROC_P5/47
  Subsystem/14(Out14) -> BCM_COM_PROC_P5/48
  Subsystem/15(Out15) -> BCM_COM_PROC_P5/49
  Subsystem/16(Out16) -> BCM_COM_PROC_P5/50
  Subsystem/17(Out17) -> BCM_COM_PROC_P5/51
  Subsystem/18(Out18) -> BCM_COM_PROC_P5/52
  Subsystem/19(Out19) -> BCM_COM_PROC_P5/53
  Subsystem/20(Out20) -> BCM_COM_PROC_P5/54
  Subsystem/21(Out21) -> BCM_COM_PROC_P5/55
  Subsystem/22(Out22) -> BCM_COM_PROC_P5/56
  Subsystem/23(Out23) -> BCM_COM_PROC_P5/57
  Subsystem/24(Out24) -> BCM_COM_PROC_P5/58
  Subsystem/25(Out25) -> BCM_COM_PROC_P5/59
  Subsystem/26(Out26) -> BCM_COM_PROC_P5/60
  Subsystem/27(Out27) -> BCM_COM_PROC_P5/61
  Subsystem/28(Out28) -> BCM_COM_PROC_P5/62
  Subsystem/29(Out29) -> BCM_COM_PROC_P5/63
  Subsystem/30(Out30) -> BCM_COM_PROC_P5/64
  Subsystem/31(Out31) -> BCM_COM_PROC_P5/65
  Subsystem/32(Out32) -> BCM_COM_PROC_P5/66
  Subsystem/33(Out33) -> BCM_COM_PROC_P5/67
  Subsystem/34(Out34) -> BCM_COM_PROC_P5/68
  Subsystem/35(Out35) -> BCM_COM_PROC_P5/69
  Subsystem/36(Out36) -> BCM_COM_PROC_P5/70
  Subsystem/37(Out37) -> BCM_COM_PROC_P5/71
  Subsystem/38(Out38) -> BCM_COM_PROC_P5/72
  Subsystem/39(Out39) -> BCM_COM_PROC_P5/73
  Subsystem/40(Out40) -> BCM_COM_PROC_P5/74
  Subsystem/41(Out41) -> BCM_COM_PROC_P5/75
  Subsystem/42(Out42) -> BCM_COM_PROC_P5/76
  Subsystem/43(Out43) -> BCM_COM_PROC_P5/77
  Subsystem/44(Out44) -> BCM_COM_PROC_P5/78
  Subsystem/45(Out45) -> BCM_COM_PROC_P5/79
  Subsystem/46(Out46) -> BCM_COM_PROC_P5/80
  Subsystem/47(Out47) -> BCM_COM_PROC_P5/81
  Subsystem/48(Out48) -> BCM_COM_PROC_P5/82
  Subsystem/49(Out49) -> BCM_COM_PROC_P5/83
  Subsystem/50(Out50) -> BCM_COM_PROC_P5/84
  Subsystem/51(Out51) -> BCM_COM_PROC_P5/85
  Subsystem/52(Out52) -> BCM_COM_PROC_P5/86
  Subsystem/53(Out53) -> BCM_COM_PROC_P5/87
  Subsystem/54(Out54) -> BCM_COM_PROC_P5/88
  Subsystem/55(Out55) -> BCM_COM_PROC_P5/89
  Subsystem/56(Out56) -> BCM_COM_PROC_P5/90
  Subsystem/57(Out57) -> BCM_COM_PROC_P5/91
  Subsystem/58(Out58) -> BCM_COM_PROC_P5/92
